simulink model "alpha10th_Order_IIR_Filter"  (R2019b)
settings: Solver=FixedStepAuto  StartTime=0.0  StopTime=testtime  RelTol=1e-3
InitFcn:
  | C2_Wideband_Test_Parameters
StopFcn:
  | Verify_C2_Wideband_Filter
undefined symbols (not defined in the file or in its folder): C2coeffs
settings Model: Creator=mblun  LastModifiedBy=t96f346
settings DataIOCC: SaveOutput=off  SaveTime=off
settings OptimizationCC: BlockReduction=off  ConditionallyExecuteInputs=off  DefaultParameterBehavior=Inlined
settings DebuggingCC: AlgebraicLoopMsg=error
settings HardwareCC: ProdBitPerPointer=32  ProdBitPerSizeT=32  ProdBitPerPtrDiffT=32  ProdLargestAtomicFloat=None  ProdIntDivRoundTo=Undefined  ProdEndianess=Unspecified  ProdWordSize=32  ProdHWDeviceType=ASIC/FPGA->ASIC/FPGA  TargetBitPerPointer=64  TargetBitPerSizeT=64  TargetBitPerPtrDiffT=64  TargetLongLongMode=on  TargetIntDivRoundTo=Zero  TargetEndianess=LittleEndian  TargetWordSize=64  TargetHWDeviceType=Custom Processor->MATLAB Host Computer  ProdEqTarget=off
settings SFSimCC: CustomCodeUndefinedFunction=UseInterfaceOnly

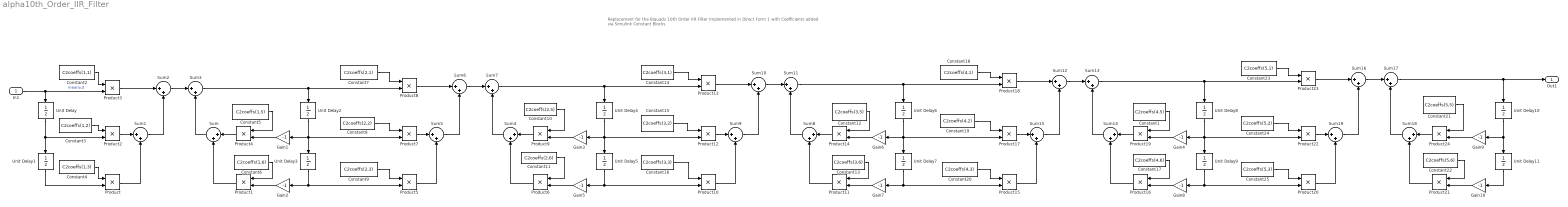
== system alpha10th_Order_IIR_Filter ==
  note: Replacement for the Biquads
      | 10th Order IIR Filter Implemented in Direct Form 1 with Coefficients added via Simulink Constant Blocks
  In1 : Inport  OutDataTypeStr=single  PortDimensions=[1 1]  SampleTime=[2.0833333333333333e-05,0]
  Constant1 : Constant  Value=C2coeffs(4,5)  OutDataTypeStr=single  SampleTime=-1
  Constant10 : Constant  Value=C2coeffs(2,5)  OutDataTypeStr=single  SampleTime=-1
  Constant11 : Constant  Value=C2coeffs(2,6)  OutDataTypeStr=single  SampleTime=-1
  Constant12 : Constant  Value=C2coeffs(3,5)  OutDataTypeStr=single  SampleTime=-1
  Constant13 : Constant  Value=C2coeffs(3,6)  OutDataTypeStr=single  SampleTime=-1
  Constant14 : Constant  Value=C2coeffs(3,1)  OutDataTypeStr=single  SampleTime=-1
  Constant15 : Constant  Value=C2coeffs(3,2)  OutDataTypeStr=single  SampleTime=-1
  Constant16 : Constant  Value=C2coeffs(3,3)  OutDataTypeStr=single  SampleTime=-1
  Constant17 : Constant  Value=C2coeffs(4,6)  OutDataTypeStr=single  SampleTime=-1
  Constant18 : Constant  Value=C2coeffs(4,1)  OutDataTypeStr=single  SampleTime=-1
  Constant19 : Constant  Value=C2coeffs(4,2)  OutDataTypeStr=single  SampleTime=-1
  Constant2 : Constant  Value=C2coeffs(1,1)  OutDataTypeStr=single  SampleTime=-1
  Constant20 : Constant  Value=C2coeffs(4,3)  OutDataTypeStr=single  SampleTime=-1
  Constant21 : Constant  Value=C2coeffs(5,5)  OutDataTypeStr=single  SampleTime=-1
  Constant22 : Constant  Value=C2coeffs(5,6)  OutDataTypeStr=single  SampleTime=-1
  Constant23 : Constant  Value=C2coeffs(5,1)  OutDataTypeStr=single  SampleTime=-1
  Constant24 : Constant  Value=C2coeffs(5,2)  OutDataTypeStr=single  SampleTime=-1
  Constant25 : Constant  Value=C2coeffs(5,3)  OutDataTypeStr=single  SampleTime=-1
  Constant3 : Constant  Value=C2coeffs(1,2)  OutDataTypeStr=single  SampleTime=-1
  Constant4 : Constant  Value=C2coeffs(1,3)  OutDataTypeStr=single  SampleTime=-1
  Constant5 : Constant  Value=C2coeffs(1,5)  OutDataTypeStr=single  SampleTime=-1
  Constant6 : Constant  Value=C2coeffs(1,6)  OutDataTypeStr=single  SampleTime=-1
  Constant7 : Constant  Value=C2coeffs(2,1)  OutDataTypeStr=single  SampleTime=-1
  Constant8 : Constant  Value=C2coeffs(2,2)  OutDataTypeStr=single  SampleTime=-1
  Constant9 : Constant  Value=C2coeffs(2,3)  OutDataTypeStr=single  SampleTime=-1
  Gain{1..10} (10 alike) : Gain  Gain=-1
  Product{,1..24} (25 alike) : Product
  Sum{,1..19} (20 alike) : Sum  Inputs=|++
  Unit Delay{,1..11} (12 alike) : UnitDelay  SampleTime=-1  HasFrameUpgradeWarning=on
  Out1 : Outport  OutDataTypeStr=single  PortDimensions=1  SampleTime=[2.0833333333333333e-05,0]
  wires:
  Sum5/1 -> Sum6/2
  Product/1 -> Sum1/2
  Constant6/1 -> Product1/1
  Sum1/1 -> Sum2/2
  Sum6/1 -> Sum7/1
  Sum2/1 -> Sum3/1
  Constant8/1 -> Product7/1
  Sum14/1 -> Sum13/2
  Constant10/1 -> Product9/1
  Product5/1 -> Sum5/2
  Product2/1 -> Sum1/1
  Gain10/1 -> Product21/2
  Constant5/1 -> Product4/1
  Unit Delay11/1 -> Gain10/1
  Constant4/1 -> Product/1
  Sum4/1 -> Sum7/2
  Constant18/1 -> Product18/1
  Constant12/1 -> Product14/1
  Product4/1 -> Sum/1
  Product17/1 -> Sum15/1
  Constant14/1 -> Product13/1
  Gain2/1 -> Product1/2
  Sum17/1 -> Out1/1, Unit Delay10/1
  Product13/1 -> Sum10/1
  Sum15/1 -> Sum12/2
  Product10/1 -> Sum9/2
  Gain3/1 -> Product9/2
  Unit Delay/1 -> Product2/2, Unit Delay1/1
  Unit Delay8/1 -> Gain4/1, Unit Delay9/1, Product22/2
  Sum19/1 -> Sum16/2
  Constant16/1 -> Product10/1
  Product9/1 -> Sum4/1
  Sum3/1 -> Product8/2, Unit Delay2/1
  Product23/1 -> Sum16/1
  Product3/1 -> Sum2/1
  Product20/1 -> Sum19/2
  Constant3/1 -> Product2/1
  Constant21/1 -> Product24/1
  Unit Delay2/1 -> Gain1/1, Unit Delay3/1, Product7/2
  Unit Delay7/1 -> Gain7/1, Product15/2
  Constant19/1 -> Product17/1
  Constant9/1 -> Product5/1
  Sum16/1 -> Sum17/1
  Constant22/1 -> Product21/1
  Constant15/1 -> Product12/1
  Product18/1 -> Sum12/1
  Constant13/1 -> Product11/1
  Sum11/1 -> Product18/2, Unit Delay6/1
  Sum/1 -> Sum3/2
  Unit Delay6/1 -> Gain6/1, Unit Delay7/1, Product17/2
  Unit Delay10/1 -> Gain9/1, Unit Delay11/1
  Gain9/1 -> Product24/2
  Gain5/1 -> Product6/2
  Product14/1 -> Sum8/1
  Sum10/1 -> Sum11/1
  Gain4/1 -> Product19/2
  Sum8/1 -> Sum11/2
  Constant17/1 -> Product16/1
  Gain1/1 -> Product4/2
  Sum9/1 -> Sum10/2
  Gain7/1 -> Product11/2
  Product6/1 -> Sum4/2
  Unit Delay1/1 -> Product/2
  Sum7/1 -> Product13/2, Unit Delay4/1
  Constant11/1 -> Product6/1
  Constant25/1 -> Product20/1
  Sum13/1 -> Product23/2, Unit Delay8/1
  Unit Delay5/1 -> Gain5/1, Product10/2
  Product16/1 -> Sum14/2
  Gain6/1 -> Product14/2
  Product7/1 -> Sum5/1
  Product22/1 -> Sum19/1
  Product15/1 -> Sum15/2
  Unit Delay3/1 -> Gain2/1, Product5/2
  Product11/1 -> Sum8/2
  Constant24/1 -> Product22/1
  Sum18/1 -> Sum17/2
  Constant20/1 -> Product15/1
  Product12/1 -> Sum9/1
  Unit Delay9/1 -> Gain8/1, Product20/2
  Unit Delay4/1 -> Gain3/1, Unit Delay5/1, Product12/2
  Constant1/1 -> Product19/1
  Product8/1 -> Sum6/1
  Gain8/1 -> Product16/2
  In1/1 -> Unit Delay/1, Product3/2  "mearout"
  Constant7/1 -> Product8/1
  Constant2/1 -> Product3/1
  Product21/1 -> Sum18/2
  Constant23/1 -> Product23/1
  Product24/1 -> Sum18/1
  Product1/1 -> Sum/2
  Product19/1 -> Sum14/1
  Sum12/1 -> Sum13/1
